simulink model "ADRC"  (R2019b)
settings: Solver=VariableStepAuto  StartTime=0.0  StopTime=10.0  RelTol=1e-3
model workspace (MAT data in the model file):
  b = Simulink.Parameter
  b.DataType = 'auto'
  b.Dimensions = [0 0]
  kp = Simulink.Parameter
  kp.DataType = 'auto'
  kp.Dimensions = [0 0]
settings Model: Creator=leony  LastModifiedBy=leonyob

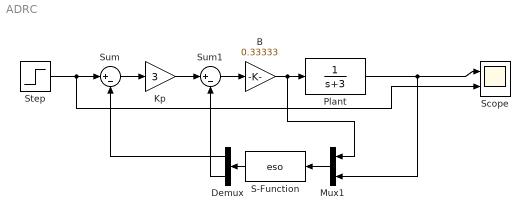
== system ADRC ==
  B : Gain  Gain=0.33333  ParamDataTypeStr=double
  Demux : Demux  Outputs=2
  Kp : Gain  Gain=3
  Mux1 : Mux  Inputs=2
  Plant : TransferFcn  Numerator=1  Denominator="[1  3]"
  S-Function : S-Function  FunctionName=eso  Parameters=b, kp  SFunctionDeploymentMode=off  EnableBusSupport=off
  Scope : Scope  NumInputPorts=2
  Step : Step  SampleTime=0
  Sum : Sum  Inputs=|+-
  Sum1 : Sum  Inputs=|+-
  wires:
  Plant/1 -> Mux1/2, Scope/1
  Mux1/1 -> S-Function/1
  S-Function/1 -> Demux/1
  Step/1 -> Scope/2, Sum/1
  Demux/1 -> Sum/2
  Sum/1 -> Kp/1
  Kp/1 -> Sum1/1
  Demux/2 -> Sum1/2
  Sum1/1 -> B/1
  B/1 -> Mux1/1, Plant/1
